simulink model "slexFMCWRFExample"  (R2018b)
settings: Solver=FixedStepDiscrete  StartTime=0.0  StopTime=32*paramFMCWRF.T  RelTol=1e-3  EnableMultiTasking=on
PreLoadFcn:
  | helperslexFMCWRFParam
undefined symbols (not defined in the file or in its folder): paramFMCWRF
libraries: simrfV2elements x10, simrfV2util1 x9, phasedenvlib x4, phasedwavlib x1, simrfV2junction1 x1, simrfV2_lib x1
CloseFcn:
  | clear paramFMCWRF
Description:
  | FMCW Radar Range Estimation
  | 
  | This model shows how to use a FMCW radar to estimate a target's range.
settings Model: Creator=The MathWorks, Inc.  LastModifiedBy=The MathWorks, Inc.
settings DataIOCC: LimitDataPoints=on  SaveFormat=Array
settings OptimizationCC: LifeSpan=inf
settings DebuggingCC: ReadBeforeWriteMsg=DisableAll  WriteAfterWriteMsg=DisableAll  WriteAfterReadMsg=DisableAll  UnderspecifiedInitializationDetection=Classic  MergeDetectMultiDrivingBlocksExec=none  SolverPrmCheckMsg=warning  MultiTaskDSMMsg=none  SFUnexpectedBacktrackingDiag=warning  SFNoUnconditionalDefaultTransitionDiag=warning  SFExecutionAtInitializationDiag=none
settings HardwareCC: ProdBitPerPointer=32  ProdBitPerSizeT=32  ProdBitPerPtrDiffT=32  ProdLargestAtomicFloat=None  ProdIntDivRoundTo=Undefined  ProdEndianess=Unspecified  ProdWordSize=32  ProdHWDeviceType=32-bit Generic
settings ModelReferenceCC: UpdateModelReferenceTargets=IfOutOfDate  PropagateSignalLabelsOutOfModel=off
settings SFSimCC: SFSimEcho=off  SimUseLocalCustomCode=off
settings RTWCC: RTWUseLocalCustomCode=off
settings CodeAppCC: StateflowObjectComments=on
settings GRTTargetCC: TargetLangStandard=C89/C90 (ANSI)  GeneratePreprocessorConditionals=Disable all
settings ConfigComp: CovMetricSettings=dw  CovHtmlReporting=on  CovSaveCumulativeToWorkspaceVar=on  CovSaveSingleToWorkspaceVar=on  CovExternalEMLEnable=off  CovSFcnEnable=off
settings SimscapeCC: SimscapeNormalizeSystem=off

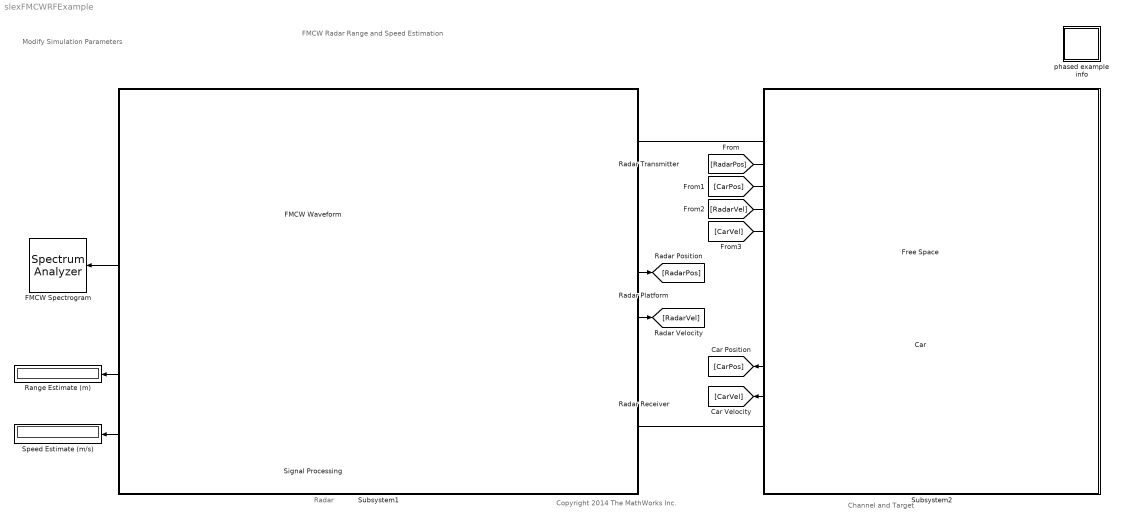
== system slexFMCWRFExample ==
  note: Copyright 2014 The MathWorks Inc.
  note: Radar
  note: Channel and Target
  note: FMCW Radar Range and Speed Estimation
  note: Modify Simulation Parameters
  Car : Subsystem
      mask Display:
      | disp('Car')
      | port_label('output',1,'Pos')
      | port_label('output',2,'Vel')
      | port_label('output',3,'Sig')
  FMCW Spectrogram : SpectrumAnalyzer
  FMCW Waveform : phasedwavlib/FMCW Waveform  SampleRate=paramFMCWRF.Fs  SweepTime=paramFMCWRF.T  SweepBandwidth=paramFMCWRF.Fs  SweepDirection=Triangle  SweepInterval=Symmetric  OutputFormat=Sweeps  NumSamples=100  NumSweeps=1  SimulateUsing=Interpreted execution
      settings: SourceProductName=Phased Array System Toolbox  SourceProductBaseCode=AR
  Free Space : phasedenvlib/Free Space  PropagationSpeed=paramFMCWRF.C  OperatingFrequency=paramFMCWRF.Fc  TwoWayPropagation=on  SampleRateFromInputCheckbox=on  SampleRate=1e6  MaximumDistanceSource=Property  MaximumDistance=10e3  MaximumNumInputSamplesSource=Auto  MaximumNumInputSamples=1000  SimulateUsing=Interpreted execution
      settings: SourceProductName=Phased Array System Toolbox  SourceProductBaseCode=AR
  Radar Platform : phasedenvlib/Motion Platform  MotionModel=Velocity  InitialPosition=paramFMCWRF.RadarPos  InitialVelocity=[ 0; 0; 0 ]  VelocitySource=Property  Velocity=paramFMCWRF.RadarVel  AccelerationSource=Property  Acceleration=[0;0;0]  CustomTrajectory=[ 0, 0, 0, 0, 0, 0, 0; 1, 0, 0, 0, 0, 0, 0 ]  ScanMode=None  InitialScanAngle=0  AzimuthSpan=[ -60, 60 ]  AzimuthScanRate=10  InitialOrientationAxes=eye( 3 )  OrientationAxesOutputPort=off  ElapsedTimeSource=Auto  SampleRateFromInputCheckbox=on  SampleRate=1e6  SimulateUsing=Interpreted execution
      settings: SourceProductName=Phased Array System Toolbox  SourceProductBaseCode=AR
  Radar Receiver : Subsystem
      mask Display:
      | disp('Receiver\nPreamp')
      | port_label('input',1,'Ref')
      | port_label('input',2,'X')
      | port_label('output',1,'Echo')
  Radar Transmitter : Subsystem
      mask Display:
      | disp('Transmitter')
      | port_label('input',1,'')
      | port_label('output',1,'Y')
      | port_label('output',2,'Ref')
  Range Estimate (m) : Display
  Signal Processing : Subsystem
      mask Display:
      | disp('Signal\nProcessing')
      | port_label('input',1,'Echo')
      | port_label('output',1,'Rng')
      | port_label('output',2,'Dechirped')
  Speed Estimate (m/s) : Display
  Subsystem1 : Subsystem
  Subsystem2 : Subsystem
  phased example info : Subsystem
      settings: OpenFcn=|
      | modelname = 'slexSimRFCosimExample';
      | helpview(fullfile(matlabroot,'help','phased','helptargets.map'),sprintf('%s',modelname));
      | clear modelname;
      mask Display: disp('Info')
  wires:
  FMCW Waveform/1 -> Radar Transmitter/1(In1), FMCW Spectrogram/1
  [RadarPos] -> Free Space/2
  [CarPos] -> Free Space/3
  [RadarVel] -> Free Space/4
  [CarVel] -> Free Space/5
  Radar Transmitter/1(Out1) -> Free Space/1
  Radar Platform/1 -> [RadarPos]
  Radar Platform/2 -> [RadarVel]
  Free Space/1 -> Car/1(In1)
  Car/1(Out1) -> [CarPos]
  Car/2(Out2) -> [CarVel]
  Radar Receiver/1(Out1) -> Signal Processing/1(In2)
  Car/3(Out3) -> Radar Receiver/2(In2)
  Radar Transmitter/2(Out2) -> Radar Receiver/1(In1)
  Signal Processing/1(Out3) -> Range Estimate (m)/1
  Signal Processing/2(Out4) -> Speed Estimate (m/s)/1

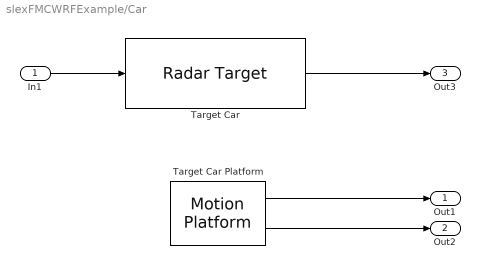
== system slexFMCWRFExample/Car ==
  In1 : Inport
  Target Car : phasedenvlib/Radar Target  EnablePolarization=off  Mode=Monostatic  MeanRCSSource=Property  ScatteringMatrixSource=Property  MeanRCS=paramFMCWRF.RCS  ScatteringMatrix=eye( 2 )  Model=Nonfluctuating  PropagationSpeed=paramFMCWRF.C  OperatingFrequency=paramFMCWRF.Fc  SeedSource=Auto  Seed=0  SimulateUsing=Interpreted execution
      settings: SourceProductName=Phased Array System Toolbox  SourceProductBaseCode=AR
  Target Car Platform : phasedenvlib/Motion Platform  MotionModel=Velocity  InitialPosition=paramFMCWRF.CarPos  InitialVelocity=[ 0; 0; 0 ]  VelocitySource=Property  Velocity=paramFMCWRF.CarVel  AccelerationSource=Property  Acceleration=[0;0;0]  CustomTrajectory=[ 0, 0, 0, 0, 0, 0, 0; 1, 0, 0, 0, 0, 0, 0 ]  ScanMode=None  InitialScanAngle=0  AzimuthSpan=[ -60, 60 ]  AzimuthScanRate=10  InitialOrientationAxes=eye( 3 )  OrientationAxesOutputPort=off  ElapsedTimeSource=Auto  SampleRateFromInputCheckbox=on  SampleRate=1e6  SimulateUsing=Interpreted execution
      settings: SourceProductName=Phased Array System Toolbox  SourceProductBaseCode=AR
  Out1 : Outport
  Out2 : Outport  Port=2
  Out3 : Outport  Port=3
  wires:
  Target Car/1 -> Out3/1
  In1/1 -> Target Car/1
  Target Car Platform/1 -> Out1/1
  Target Car Platform/2 -> Out2/1

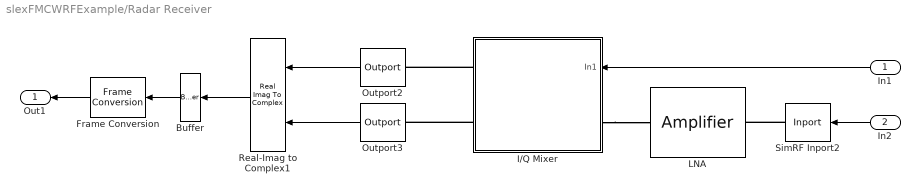
== system slexFMCWRFExample/Radar Receiver ==
  In1 : Inport
  In2 : Inport  Port=2
  Buffer : Buffer  N=paramFMCWRF.Fs*paramFMCWRF.T
  Frame Conversion : FrameConversion  OutFrame=Sample-based
  I/Q Mixer : Subsystem
  LNA : simrfV2elements/Amplifier  classname=amplifier  DataSource=Data file  File=unitygain.s2p  Paramtype=S-parameters  Sparam=[0 0;1 0]  SparamFreq=1e9 Hz  SparamZ0=50  Residues=0  Poles=0  DF={0 0; 1 0}  Source_linear_gain=Available power gain  linear_gain=paramFMCWRF.lna_gain dB  Zin=50  Zout=50  Source_Poly=Even and odd order  Poly_Coeffs=[0 1]  IPType=Input  IP2=inf dBm  IP3=paramFMCWRF.lna_ip3 dBm  P1dB=inf dBm  Psat=inf dBm  Gcomp=inf dBm  InternalGrounding=on  SourceFreq=Extracted from data source  PlotFreq=1 Hz  PlotType=X-Y plane  YParam1=S11  YFormat1=Magnitude (decibels)  YParam2=None  YFormat2=Magnitude (decibels)  YOption=Linear  XOption=Linear  SparamRepresentation=Time domain (rationalfit)  FitTol=-40  FitOpt=Fit individually  AutoImpulseLength=off  ImpulseLength=0 s  MagModeling=off  AddNoise=on  NoiseType=Noise figure  NoiseDist=White  NF=paramFMCWRF.lna_nf  MinNF=0  Gopt=0  RN=0  CarrierFreq=0 Hz  NoiseAutoImpulseLength=on  NoiseImpulseLength=1e-10 s  SpecifyOpFreq=off  OpFreq=0 Hz
      settings: SourceProductName=RF Blockset  SourceProductBaseCode=RB
  Outport2 : simrfV2util1/Outport  SensorType=Power  OutputFormat=Real Passband  CarrierFreq=0 Hz  ZL=100  InternalGrounding=on  StepSize=-1 s  AutoStep=off
      settings: SourceProductName=RF Blockset  SourceProductBaseCode=RB
  Outport3 : simrfV2util1/Outport  SensorType=Power  OutputFormat=Real Passband  CarrierFreq=0 Hz  ZL=100  InternalGrounding=on  StepSize=-1 s  AutoStep=off
      settings: SourceProductName=RF Blockset  SourceProductBaseCode=RB
  Real-Imag to Complex1 : RealImagToComplex
  SimRF Inport2 : simrfV2util1/Inport  SimulinkInputSignalType=Power  CarrierFreq=paramFMCWRF.Fc Hz  ZS=50  InternalGrounding=on
      settings: SourceProductName=RF Blockset  SourceProductBaseCode=RB
  Out1 : Outport
  wires:
  Real-Imag to Complex1/1 -> Buffer/1
  Outport2/1 -> Real-Imag to Complex1/1
  Outport3/1 -> Real-Imag to Complex1/2
  Buffer/1 -> Frame Conversion/1
  Frame Conversion/1 -> Out1/1
  In1/1 -> I/Q Mixer/1(In1)
  In2/1 -> SimRF Inport2/1
  connections:
  SimRF Inport2/RConn1 -- LNA/LConn1
  I/Q Mixer/RConn1 -- Outport2/LConn1
  I/Q Mixer/RConn2 -- Outport3/LConn1
  I/Q Mixer/LConn1 -- LNA/RConn1

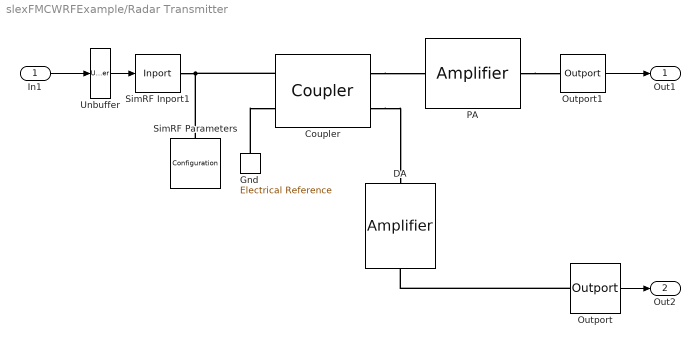
== system slexFMCWRFExample/Radar Transmitter ==
  In1 : Inport
  "Coupler " : simrfV2junction1/Coupler  classname=couplers  DataSource=Network-parameters  NumPorts=4  DeviceCirculator=Circulator clockwise  DeviceDivider=T power divider  DeviceCoupler=Hybrid quadrature (90 deg)  Paramtype=S-parameters  Sparam=[0 0 1; 1 0 0; 0 1 0]  SparamFreq=1e9 Hz  SparamZ0=50  Phase12=0  Phase33=0  Alpha=0  Coupling=0  Directivity=inf  InsertionLoss=inf  ReturnLoss=inf  InternalGrounding=on  SparamRepresentation=Frequency domain  FitOpt=Share all poles  FitTol=-40
      settings: SourceProductName=RF Blockset  SourceProductBaseCode=RB
  DA : simrfV2elements/Amplifier  classname=amplifier  DataSource=Data file  File=unitygain.s2p  Paramtype=S-parameters  Sparam=[0 0;1 0]  SparamFreq=1e9 Hz  SparamZ0=50  Residues=0  Poles=0  DF={0 0; 1 0}  Source_linear_gain=Available power gain  linear_gain=paramFMCWRF.da_gain dB  Zin=50  Zout=50  Source_Poly=Even and odd order  Poly_Coeffs=[0 1]  IPType=Output  IP2=inf dBm  IP3=inf dBm  P1dB=inf dBm  Psat=inf dBm  Gcomp=inf dBm  InternalGrounding=on  SourceFreq=Extracted from data source  PlotFreq=1 Hz  PlotType=X-Y plane  YParam1=S11  YFormat1=Magnitude (decibels)  YParam2=None  YFormat2=Magnitude (decibels)  YOption=Linear  XOption=Linear  SparamRepresentation=Time domain (rationalfit)  FitTol=-40  FitOpt=Fit individually  AutoImpulseLength=off  ImpulseLength=0 s  MagModeling=off  AddNoise=on  NoiseType=Noise figure  NoiseDist=White  NF=paramFMCWRF.da_nf  MinNF=0  Gopt=0  RN=0  CarrierFreq=0 Hz  NoiseAutoImpulseLength=on  NoiseImpulseLength=1e-10 s  SpecifyOpFreq=off  OpFreq=0 Hz
      settings: SourceProductName=RF Blockset  SourceProductBaseCode=RB
  Gnd : simrfV2_lib/Elements/Electrical Reference
  Outport : simrfV2util1/Outport  SensorType=Ideal voltage  OutputFormat=Complex Baseband  CarrierFreq=paramFMCWRF.Fc Hz  ZL=Inf  InternalGrounding=on  StepSize=1e-6 s  AutoStep=on
      settings: SourceProductName=RF Blockset  SourceProductBaseCode=RB
  Outport1 : simrfV2util1/Outport  SensorType=Power  OutputFormat=Complex Baseband  CarrierFreq=paramFMCWRF.Fc Hz  ZL=50  InternalGrounding=on  StepSize=-1 s  AutoStep=off
      settings: SourceProductName=RF Blockset  SourceProductBaseCode=RB
  PA : simrfV2elements/Amplifier  classname=amplifier  DataSource=Data file  File=unitygain.s2p  Paramtype=S-parameters  Sparam=[0 0;1 0]  SparamFreq=1e9 Hz  SparamZ0=50  Residues=0  Poles=0  DF={0 0; 1 0}  Source_linear_gain=Available power gain  linear_gain=paramFMCWRF.pa_gain dB  Zin=50  Zout=50  Source_Poly=Odd order  Poly_Coeffs=[0 1]  IPType=Input  IP2=inf dBm  IP3=paramFMCWRF.pa_ip3 dBm  P1dB=paramFMCWRF.pa_1dBc dBm  Psat=paramFMCWRF.pa_psat dBm  Gcomp=inf dBm  InternalGrounding=on  SourceFreq=Extracted from data source  PlotFreq=1 Hz  PlotType=X-Y plane  YParam1=S11  YFormat1=Magnitude (decibels)  YParam2=None  YFormat2=Magnitude (decibels)  YOption=Linear  XOption=Linear  SparamRepresentation=Time domain (rationalfit)  FitTol=-40  FitOpt=Fit individually  AutoImpulseLength=off  ImpulseLength=0 s  MagModeling=off  AddNoise=on  NoiseType=Noise figure  NoiseDist=White  NF=paramFMCWRF.pa_nf  MinNF=0  Gopt=0  RN=0  CarrierFreq=0 Hz  NoiseAutoImpulseLength=on  NoiseImpulseLength=1e-10 s  SpecifyOpFreq=off  OpFreq=0 Hz
      settings: SourceProductName=RF Blockset  SourceProductBaseCode=RB
  SimRF Inport1 : simrfV2util1/Inport  SimulinkInputSignalType=Power  CarrierFreq=paramFMCWRF.Fc Hz  ZS=50  InternalGrounding=on
      settings: SourceProductName=RF Blockset  SourceProductBaseCode=RB
  SimRF Parameters : simrfV2util1/Configuration  AutoFreq=off  Tones=77 GHz  Harmonics=paramFMCWRF.HarmonicOrder  NormalizeCarrierPower=off  SolverType=Auto  UseCCode=on  StepSize=1/paramFMCWRF.Fs s  AddNoise=on  defaultRNG=on  Seed=0  Temperature=paramFMCWRF.NoiseTemp K  SolverDelFlag=0  AbsTol=1e-6  RelTol=1e-3  MaxIter=10  ErrorEstimationType=2-norm over all variables  EnableInterpFilter=off  HiddenFIRfilterControllerParam=off
      settings: SourceProductName=RF Blockset  SourceProductBaseCode=RB
  Unbuffer : Unbuffer
  Out1 : Outport
  Out2 : Outport  Port=2
  wires:
  Unbuffer/1 -> SimRF Inport1/1
  In1/1 -> Unbuffer/1
  Outport1/1 -> Out1/1
  Outport/1 -> Out2/1
  connections:
  PA/RConn1 -- Outport1/LConn1
  "Coupler "/RConn2 -- DA/LConn1
  "Coupler "/RConn1 -- PA/LConn1
  SimRF Inport1/RConn1 -- SimRF Parameters/LConn1 -- "Coupler "/LConn1
  Gnd/LConn1 -- "Coupler "/LConn2
  Outport/LConn1 -- DA/RConn1

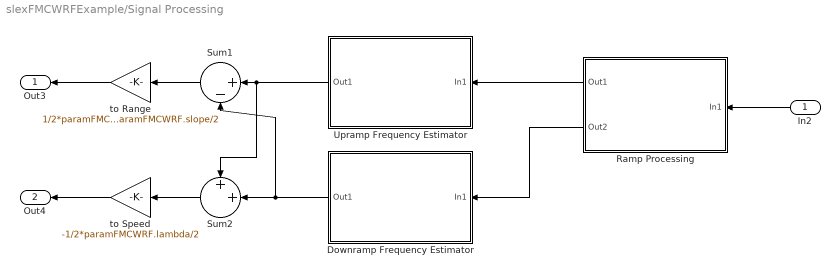
== system slexFMCWRFExample/Signal Processing ==
  In2 : Inport
  Downramp Frequency Estimator : Subsystem  mask(Range Estimator){N=2048*8}
      mask prompts: N "Number of FFT Points"
      mask help: Compute periodogram of the incoming signal, find the beat frequency, and convert the beat frequency to the range estimate.
      mask Display:
      | disp('Downramp Beat\nFrequency')
      | port_label('input',1,'X')
      | port_label('output',1,'f_b','TexMode','on')
  Ramp Processing : Subsystem  mask{N=2}
      mask prompts: N "Number of Pulses"
      mask Display:
      | disp('Pulse\nIntegration')
      | port_label('output',1,'Upramp')
      | port_label('output',2,'Downramp')
  Sum1 : Sum  Inputs=|+-
  Sum2 : Sum  Inputs=++|
  Upramp Frequency Estimator : Subsystem  mask(Range Estimator){N=2048*8}
      mask prompts: N "Number of FFT Points"
      mask help: Compute periodogram of the incoming signal, find the beat frequency, and convert the beat frequency to the range estimate.
      mask Display:
      | disp('Upramp Beat\nFrequency')
      | port_label('input',1,'X')
      | port_label('output',1,'f_b','TexMode','on')
  to Range : Gain  Gain=1/2*paramFMCWRF.C/paramFMCWRF.slope/2
  to Speed : Gain  Gain=-1/2*paramFMCWRF.lambda/2
  Out3 : Outport
  Out4 : Outport  Port=2
  wires:
  Ramp Processing/1(Out1) -> Upramp Frequency Estimator/1(In1)
  Ramp Processing/2(Out2) -> Downramp Frequency Estimator/1(In1)
  Downramp Frequency Estimator/1(Out1) -> Sum2/2, Sum1/2
  Upramp Frequency Estimator/1(Out1) -> Sum2/1, Sum1/1
  Sum1/1 -> to Range/1
  to Range/1 -> Out3/1
  Sum2/1 -> to Speed/1
  to Speed/1 -> Out4/1
  In2/1 -> Ramp Processing/1(In1)

== system slexFMCWRFExample/Subsystem1 ==

== system slexFMCWRFExample/Subsystem2 ==

== system slexFMCWRFExample/phased example info ==

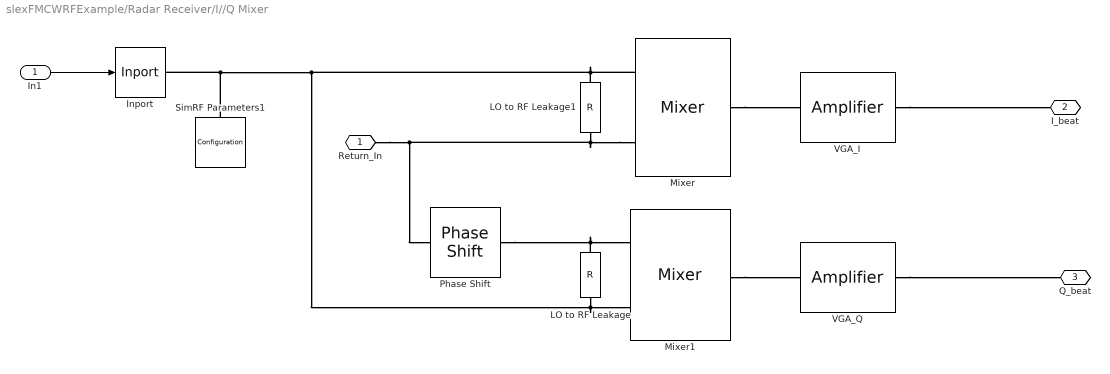
== system slexFMCWRFExample/Radar Receiver/I//Q Mixer ==
  In1 : Inport
  Inport : simrfV2util1/Inport  SimulinkInputSignalType=Ideal voltage  CarrierFreq=paramFMCWRF.Fc Hz  ZS=0  InternalGrounding=on
      settings: SourceProductName=RF Blockset  SourceProductBaseCode=RB
  LO to RF Leakage : simrfV2elements/R  classname=resistor  Resistance=paramFMCWRF.Risolation Ohm  AddNoise=off
      settings: SourceProductName=RF Blockset  SourceProductBaseCode=RB
  LO to RF Leakage1 : simrfV2elements/R  classname=resistor  Resistance=paramFMCWRF.Risolation Ohm  AddNoise=off
      settings: SourceProductName=RF Blockset  SourceProductBaseCode=RB
  Mixer : simrfV2elements/Mixer  classname=mixer  Source_linear_gain=Available power gain  linear_gain=paramFMCWRF.mix_loss dB  Zin=100  Zout=100  ZLO=100  Source_Poly=Even and odd order  Poly_Coeffs=[0 1]  IPType=Input  IP2=paramFMCWRF.mix_ip2 dBm  IP3=inf dBm  P1dB=Inf dBm  Psat=Inf dBm  Gcomp=Inf dBm  NF=paramFMCWRF.mix_nf  InternalGrounding=on
      settings: SourceProductName=RF Blockset  SourceProductBaseCode=RB
  Mixer1 : simrfV2elements/Mixer  classname=mixer  Source_linear_gain=Available power gain  linear_gain=paramFMCWRF.mix_loss dB  Zin=100  Zout=100  ZLO=100  Source_Poly=Even and odd order  Poly_Coeffs=[0 1]  IPType=Input  IP2=paramFMCWRF.mix_ip2 dBm  IP3=Inf dBm  P1dB=Inf dBm  Psat=Inf dBm  Gcomp=Inf dBm  NF=paramFMCWRF.mix_nf  InternalGrounding=on
      settings: SourceProductName=RF Blockset  SourceProductBaseCode=RB
  Phase Shift : simrfV2elements/Phase Shift  PhaseShift=90 deg  InternalGrounding=on
      settings: SourceProductName=RF Blockset  SourceProductBaseCode=RB
  SimRF Parameters1 : simrfV2util1/Configuration  AutoFreq=off  Tones=77 GHz  Harmonics=paramFMCWRF.HarmonicOrder  NormalizeCarrierPower=off  SolverType=Auto  UseCCode=on  StepSize=1/paramFMCWRF.Fs s  AddNoise=on  defaultRNG=on  Seed=0  Temperature=paramFMCWRF.NoiseTemp K  SolverDelFlag=0  AbsTol=1e-6  RelTol=1e-3  MaxIter=10  ErrorEstimationType=2-norm over all variables  EnableInterpFilter=off  HiddenFIRfilterControllerParam=off
      settings: SourceProductName=RF Blockset  SourceProductBaseCode=RB
  VGA_I : simrfV2elements/Amplifier  classname=amplifier  DataSource=Data file  File=unitygain.s2p  Paramtype=S-parameters  Sparam=[0 0;1 0]  SparamFreq=1e9 Hz  SparamZ0=50  Residues=0  Poles=0  DF={0 0; 1 0}  Source_linear_gain=Available power gain  linear_gain=paramFMCWRF.vga_gain dB  Zin=100  Zout=100  Source_Poly=Even and odd order  Poly_Coeffs=[0 1]  IPType=Output  IP2=inf dBm  IP3=inf dBm  P1dB=inf dBm  Psat=inf dBm  Gcomp=inf dBm  InternalGrounding=on  SourceFreq=Extracted from data source  PlotFreq=1 Hz  PlotType=X-Y plane  YParam1=S11  YFormat1=Magnitude (decibels)  YParam2=None  YFormat2=Magnitude (decibels)  YOption=Linear  XOption=Linear  SparamRepresentation=Time domain (rationalfit)  FitTol=-40  FitOpt=Fit individually  AutoImpulseLength=off  ImpulseLength=0 s  MagModeling=off  AddNoise=on  NoiseType=Noise figure  NoiseDist=White  NF=paramFMCWRF.vga_nf  MinNF=0  Gopt=0  RN=0  CarrierFreq=0 Hz  NoiseAutoImpulseLength=on  NoiseImpulseLength=1e-10 s  SpecifyOpFreq=off  OpFreq=0 Hz
      settings: SourceProductName=RF Blockset  SourceProductBaseCode=RB
  VGA_Q : simrfV2elements/Amplifier  classname=amplifier  DataSource=Data file  File=unitygain.s2p  Paramtype=S-parameters  Sparam=[0 0;1 0]  SparamFreq=1e9 Hz  SparamZ0=50  Residues=0  Poles=0  DF={0 0; 1 0}  Source_linear_gain=Available power gain  linear_gain=paramFMCWRF.vga_gain dB  Zin=100  Zout=100  Source_Poly=Even and odd order  Poly_Coeffs=[0 1]  IPType=Output  IP2=inf dBm  IP3=inf dBm  P1dB=inf dBm  Psat=inf dBm  Gcomp=inf dBm  InternalGrounding=on  SourceFreq=Extracted from data source  PlotFreq=1 Hz  PlotType=X-Y plane  YParam1=S11  YFormat1=Magnitude (decibels)  YParam2=None  YFormat2=Magnitude (decibels)  YOption=Linear  XOption=Linear  SparamRepresentation=Time domain (rationalfit)  FitTol=-40  FitOpt=Fit individually  AutoImpulseLength=off  ImpulseLength=0 s  MagModeling=off  AddNoise=on  NoiseType=Noise figure  NoiseDist=White  NF=paramFMCWRF.vga_nf  MinNF=0  Gopt=0  RN=0  CarrierFreq=0 Hz  NoiseAutoImpulseLength=on  NoiseImpulseLength=1e-10 s  SpecifyOpFreq=off  OpFreq=0 Hz
      settings: SourceProductName=RF Blockset  SourceProductBaseCode=RB
  Return_In : PMIOPort  Side=Left
  I_beat : PMIOPort  Port=2  Side=Right
  Q_beat : PMIOPort  Port=3  Side=Right
  wires:
  In1/1 -> Inport/1
  connections:
  Mixer/RConn1 -- VGA_I/LConn1
  Mixer1/RConn1 -- VGA_Q/LConn1
  LO to RF Leakage/LConn1 -- Phase Shift/RConn1 -- Mixer1/LConn2
  Mixer/LConn2 -- Return_In/RConn1 -- Phase Shift/LConn1 -- LO to RF Leakage1/RConn1
  VGA_I/RConn1 -- I_beat/RConn1
  VGA_Q/RConn1 -- Q_beat/RConn1
  Inport/RConn1 -- Mixer/LConn1 -- LO to RF Leakage1/LConn1 -- LO to RF Leakage/RConn1 -- Mixer1/LConn1 -- SimRF Parameters1/LConn1

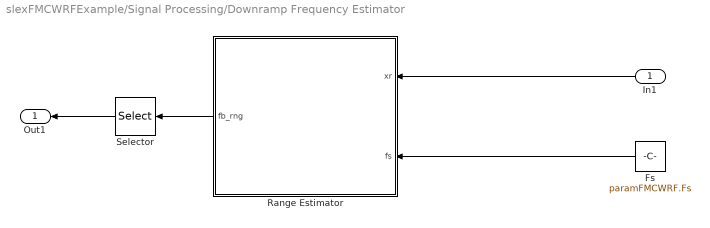
== system slexFMCWRFExample/Signal Processing/Downramp Frequency Estimator ==
  In1 : Inport
  Fs : Constant  Value=paramFMCWRF.Fs
  Range Estimator : MATLAB Function  TreatAsAtomicUnit=on
  Selector : Selector  InputPortWidth=2  IndexOptions=Index vector (dialog)  Indices=1  OutputSizes=1
  Out1 : Outport
  wires:
  Fs/1 -> Range Estimator/2(fs)
  In1/1 -> Range Estimator/1(xr)
  Range Estimator/1(fb_rng) -> Selector/1
  Selector/1 -> Out1/1

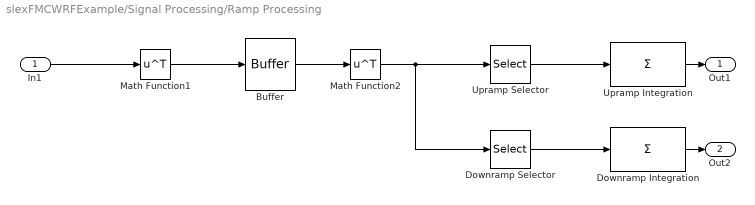
== system slexFMCWRFExample/Signal Processing/Ramp Processing ==
  In1 : Inport
  Buffer : Buffer  N=N
  Downramp Integration : Sum  Inputs=+  CollapseMode=Specified dimension  CollapseDim=2
  Downramp Selector : Selector  NumberOfDimensions=2  InputPortWidth=3  IndexOptions=Select all,Index vector (dialog)  Indices=[1 3],2:2:2  OutputSizes=1,1
  Math Function1 : Math  Operator=transpose  OutputSignalType=complex  SaturateOnIntegerOverflow=on
  Math Function2 : Math  Operator=transpose  OutputSignalType=complex  SaturateOnIntegerOverflow=on
  Upramp Integration : Sum  Inputs=+  CollapseMode=Specified dimension  CollapseDim=2
  Upramp Selector : Selector  NumberOfDimensions=2  InputPortWidth=3  IndexOptions=Select all,Index vector (dialog)  Indices=[1 3],1:2:2  OutputSizes=1,1
  Out1 : Outport
  Out2 : Outport  Port=2
  wires:
  In1/1 -> Math Function1/1
  Math Function1/1 -> Buffer/1
  Buffer/1 -> Math Function2/1
  Math Function2/1 -> Downramp Selector/1, Upramp Selector/1
  Upramp Selector/1 -> Upramp Integration/1
  Downramp Selector/1 -> Downramp Integration/1
  Upramp Integration/1 -> Out1/1
  Downramp Integration/1 -> Out2/1

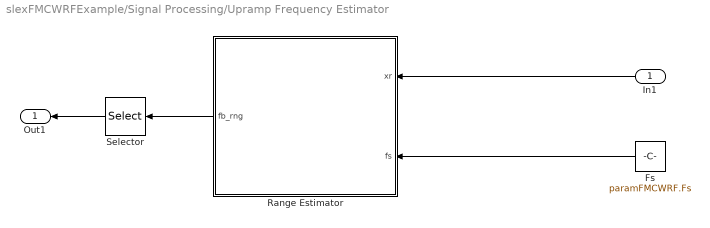
== system slexFMCWRFExample/Signal Processing/Upramp Frequency Estimator ==
  In1 : Inport
  Fs : Constant  Value=paramFMCWRF.Fs
  Range Estimator : MATLAB Function  TreatAsAtomicUnit=on
  Selector : Selector  InputPortWidth=2  IndexOptions=Index vector (dialog)  Indices=1  OutputSizes=1
  Out1 : Outport
  wires:
  Range Estimator/1(fb_rng) -> Selector/1
  In1/1 -> Range Estimator/1(xr)
  Fs/1 -> Range Estimator/2(fs)
  Selector/1 -> Out1/1

== matlab function slexFMCWRFExample/Signal Processing/Downramp Frequency Estimator/Range Estimator ==
  data: xr input; fb_rng output; fs input; N parameter
function fb_rng = fcn(xr,fs,N)
%#codegen

f = fs*(-0.5+(0:N-1)/N);
P = abs(fftshift(fft(xr,N))).^2;
[~,idx] = findpeaks(P,'NPeaks',2,'SortStr','descend');
if ~isempty(idx)
    idx2 = idx(1:2);
    fb_rng = f(idx2);
else
    fb_rng = zeros(1,2);
end

== matlab function slexFMCWRFExample/Signal Processing/Upramp Frequency Estimator/Range Estimator ==
  data: xr input; fb_rng output; fs input; N parameter
function fb_rng = fcn(xr,fs,N)
%#codegen

f = fs*(-0.5+(0:N-1)/N);
P = abs(fftshift(fft(xr,N))).^2;
[~,idx] = findpeaks(P,'NPeaks',2,'SortStr','descend');
if ~isempty(idx)
    idx2 = idx(1:2);
    fb_rng = f(idx2);
else
    fb_rng = zeros(1,2);
end
